simulink model "DriveCtrlModeBase2012"  (R2012a)
settings: Solver=FixedStepDiscrete  SolverMode=SingleTasking  StartTime=0.0  StopTime=10.0  FixedStep=1e-4  RelTol=1e-3
settings Model: CovMetricSettings=dwe  CovHtmlReporting=off  covSaveCumulativeToWorkspaceVar=off  CovSaveSingleToWorkspaceVar=off  CovExternalEMLEnable=on  Creator=F001456D  LastModifiedBy=C000874D
settings DataIOCC: SaveFormat=StructureWithTime  ReturnWorkspaceOutputs=off
settings OptimizationCC: LifeSpan=inf  SimCompilerOptimization=Off
settings DebuggingCC: InheritedTsInSrcMsg=none  FcnCallInpInsideContextMsg=Enable All  RootOutportRequireBusObject=error  StrictBusMsg=ErrorOnBusTreatedAsVector
settings HardwareCC: ProdBitPerPointer=32  ProdLargestAtomicInteger=Long  ProdWordSize=32  ProdHWDeviceType=ARM Compatible->ARM 7
settings SFSimCC: SimUseLocalCustomCode=off
settings RTWCC: SystemTargetFile=MTRealTime_ZYNQ.tlc  TemplateMakefile=MTRealTime_ZYNQ.tmf  Description=MT RealTime ZYNQ Target  RTWUseLocalCustomCode=off  RTWCompilerOptimization=Off
settings STFCustomTargetCC: CodeReplacementLibrary=C99 (ISO)  SystemTargetFile=MTRealTime_ZYNQ.tlc
settings GRTTargetCC: CodeReplacementLibrary=C99 (ISO)  ParMdlRefBuildCompliant=off  CompOptLevelCompliant=off  ConcurrentExecutionCompliant=off  CombineOutputUpdateFcns=off  MatFileLogging=off  CPPClassGenCompliant=off  GRTInterface=on
settings SimscapeCC: SimscapeNormalizeSystem=off

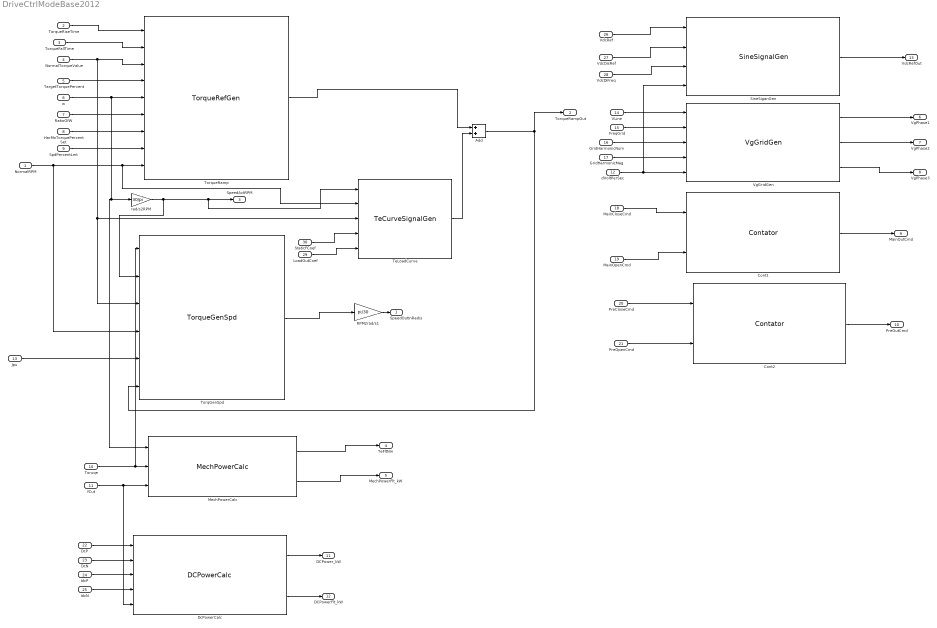
== system DriveCtrlModeBase2012 ==
  NormalRPM : Inport
  TorqueRiseTime : Inport  Port=2
  TorqueFallTime : Inport  Port=3
  NormalTorqueValue : Inport  Port=4
  TargetTorquePercent : Inport  Port=5
  w : Inport  Port=6
  RatioOfW : Inport  Port=7
  HarMoTorquePercentSet : Inport  Port=8
  SpdPercentLmt : Inport  Port=9
  Toruqe : Inport  Port=10
  fCut : Inport  Port=11
  dVoltPerSec : Inport  Port=12
  Jpu : Inport  Port=13
  VLine : Inport  Port=14
  FreqGrid : Inport  Port=15
  GridHarmonicNum : Inport  Port=16
  GridHarmonicMag : Inport  Port=17
  MainCloseCmd : Inport  Port=18
  MainOpenCmd : Inport  Port=19
  PreCloseCmd : Inport  Port=20
  PreOpenCmd : Inport  Port=21
  DcP : Inport  Port=22
  DcN : Inport  Port=23
  IdcP : Inport  Port=24
  IdcN : Inport  Port=25
  VdcRef : Inport  Port=26
  VdcDisRef : Inport  Port=27
  VdcDiFreq : Inport  Port=28
  LoadOutCoef : Inport  Port=29
  StaticFCoef : Inport  Port=30
  Add : Sum
  Cont1 : S-Function  InitFcn=try, set_param(gcb,'FunctionName','Contator'), end  FunctionName=Contator  SFunctionModules=Contator_wrapper  SFunctionDeploymentMode=off  EnableBusSupport=off  mask(S-Function Builder){}
      mask help: Simulink:masks:SFunctionBuilder_MD
      mask init:
      | val = [[.9  0.75 0.75 1 1 .9 .9 1]',[1 1 0.75 0.75 .9 .9 1 .9]'];try , sys = get_param(gcb,'SfunBuilderFcnName');if isempty(sys), sys = get_param(gcb,'FunctionName'); end,catch, sys = get_param(gcb,'FunctionName'); end
      settings: CopyFcn=set_param(gcbh,'LinkStatus','none')  PreSaveFcn=try, set_param(gcb,'FunctionName','Contator'), end  OpenFcn=sfunctionwizard(gcbh)
      mask Display: plot(val(:,1),val(:,2)),disp(sys), port_label('input',1,'CloseCmd'), port_label('input',2,'OpenCmd'), port_label('output',1,'ConCmd')
  Cont2 : S-Function  InitFcn=try, set_param(gcb,'FunctionName','Contator'), end  FunctionName=Contator  SFunctionModules=Contator_wrapper  SFunctionDeploymentMode=off  EnableBusSupport=off  mask(S-Function Builder){}
      mask help: Simulink:masks:SFunctionBuilder_MD
      mask init: same as DriveCtrlModeBase2012/Cont1
      settings: CopyFcn=set_param(gcbh,'LinkStatus','none')  PreSaveFcn=try, set_param(gcb,'FunctionName','Contator'), end  OpenFcn=sfunctionwizard(gcbh)
      mask Display: plot(val(:,1),val(:,2)),disp(sys), port_label('input',1,'CloseCmd'), port_label('input',2,'OpenCmd'), port_label('output',1,'ConCmd')
  DcPowerCalc : S-Function  InitFcn=try, set_param(gcb,'FunctionName','DCPowerCalc'), end  FunctionName=DCPowerCalc  SFunctionModules=DCPowerCalc_wrapper  SFunctionDeploymentMode=off  EnableBusSupport=off  mask(S-Function Builder){}
      mask help: Simulink:masks:SFunctionBuilder_MD
      mask init: same as DriveCtrlModeBase2012/Cont1
      settings: CopyFcn=set_param(gcbh,'LinkStatus','none')  PreSaveFcn=try, set_param(gcb,'FunctionName','DCPowerCalc'), end  OpenFcn=sfunctionwizard(gcbh)
      mask Display: plot(val(:,1),val(:,2)),disp(sys), port_label('input',1,'VdcP'), port_label('input',2,'VdcN'), port_label('input',3,'IdcP'), port_label('input',4,'IdcN'), port_label('input',5,'fCut'), port_label('output',1,'DCPower_kW'), port_label('output',2,'DCPowerFlt_kW')
  MechPowerCalc : S-Function  InitFcn=try, set_param(gcb,'FunctionName','MechPowerCalc'), end  FunctionName=MechPowerCalc  SFunctionModules=MechPowerCalc_wrapper  SFunctionDeploymentMode=off  EnableBusSupport=off  mask(S-Function Builder){}
      mask help: Simulink:masks:SFunctionBuilder_MD
      mask init: same as DriveCtrlModeBase2012/Cont1
      settings: CopyFcn=set_param(gcbh,'LinkStatus','none')  PreSaveFcn=try, set_param(gcb,'FunctionName','MechPowerCalc'), end  OpenFcn=sfunctionwizard(gcbh)
      mask Display: plot(val(:,1),val(:,2)),disp(sys), port_label('input',1,'Wm'), port_label('input',2,'Torque'), port_label('input',3,'fCut'), port_label('output',1,'MechPower_kW'), port_label('output',2,'MechPowerFlt_kW')
  RPM2rad/s1 : Gain  Gain=pi/30
  SineSiganGen : S-Function  InitFcn=try, set_param(gcb,'FunctionName','SineSignalGen'), end  FunctionName=SineSignalGen  SFunctionModules=SineSignalGen_wrapper  SFunctionDeploymentMode=off  EnableBusSupport=off  mask(S-Function Builder){}
      mask help: Simulink:masks:SFunctionBuilder_MD
      mask init: same as DriveCtrlModeBase2012/Cont1
      settings: CopyFcn=set_param(gcbh,'LinkStatus','none')  PreSaveFcn=try, set_param(gcb,'FunctionName','SineSignalGen'), end  OpenFcn=sfunctionwizard(gcbh)
      mask Display: plot(val(:,1),val(:,2)),disp(sys), port_label('input',1,'DCMag'), port_label('input',2,'ACMag'), port_label('input',3,'Freq'), port_label('input',4,'dVoltPerSec'), port_label('output',1,'SineOut')
  TeLoadCurve : S-Function  InitFcn=try, set_param(gcb,'FunctionName','TeCurveSignalGen'), end  FunctionName=TeCurveSignalGen  SFunctionModules=TeCurveSignalGen_wrapper  SFunctionDeploymentMode=off  EnableBusSupport=off  mask(S-Function Builder){}
      mask help: Simulink:masks:SFunctionBuilder_MD
      mask init: same as DriveCtrlModeBase2012/Cont1
      settings: CopyFcn=set_param(gcbh,'LinkStatus','none')  PreSaveFcn=try, set_param(gcb,'FunctionName','TeCurveSignalGen'), end  OpenFcn=sfunctionwizard(gcbh)
      mask Display: plot(val(:,1),val(:,2)),disp(sys), port_label('input',1,'nrpm'), port_label('input',2,'NormRpm'), port_label('input',3,'TeNorm'), port_label('input',4,'StaticFCoef'), port_label('input',5,'KpLoadCurve'), port_label('output',1,'TLCurveOut')
  TorqGenSpd : S-Function  InitFcn=try, set_param(gcb,'FunctionName','TorqueGenSpd'), end  FunctionName=TorqueGenSpd  SFunctionModules=TorqueGenSpd_wrapper  SFunctionDeploymentMode=off  EnableBusSupport=off  mask(S-Function Builder){}
      mask help: Simulink:masks:SFunctionBuilder_MD
      mask init: same as DriveCtrlModeBase2012/Cont1
      settings: CopyFcn=set_param(gcbh,'LinkStatus','none')  PreSaveFcn=try, set_param(gcb,'FunctionName','TorqueGenSpd'), end  OpenFcn=sfunctionwizard(gcbh)
      mask Display: plot(val(:,1),val(:,2)),disp(sys), port_label('input',1,'TorqMotor'), port_label('input',2,'SpdAct'), port_label('input',3,'TorqBase'), port_label('input',4,'SpdBase'), port_label('input',5,'Jpu'), port_label('input',6,'TorqLoad'), port_label('output',1,'SpdSetOut')
  TorqueRamp : S-Function  InitFcn=try, set_param(gcb,'FunctionName','TorqueRefGen'), end  FunctionName=TorqueRefGen  SFunctionModules=TorqueRefGen_wrapper  SFunctionDeploymentMode=off  EnableBusSupport=off  mask(S-Function Builder){}
      mask help: Simulink:masks:SFunctionBuilder_MD
      mask init: same as DriveCtrlModeBase2012/Cont1
      settings: CopyFcn=set_param(gcbh,'LinkStatus','none')  PreSaveFcn=try, set_param(gcb,'FunctionName','TorqueRefGen'), end  OpenFcn=sfunctionwizard(gcbh)
      mask Display: plot(val(:,1),val(:,2)),disp(sys), port_label('input',1,'RiseTime'), port_label('input',2,'FallTime'), port_label('input',3,'NormalValue'), port_label('input',4,'DestValuePercent'), port_label('input',5,'w'), port_label('input',6,'RatioOfW'), port_label('input',7,'HarmoTorquePercent'), port_label('input',8,'SpdPercentLmt'), port_label('input',9,'RPMNorm'), port_label('output',1,'RampOut')
  VgGridGen : S-Function  InitFcn=try, set_param(gcb,'FunctionName','VgGridGen'), end  FunctionName=VgGridGen  SFunctionModules=VgGridGen_wrapper  SFunctionDeploymentMode=off  EnableBusSupport=off  mask(S-Function Builder){}
      mask help: Simulink:masks:SFunctionBuilder_MD
      mask init: same as DriveCtrlModeBase2012/Cont1
      settings: CopyFcn=set_param(gcbh,'LinkStatus','none')  PreSaveFcn=try, set_param(gcb,'FunctionName','VgGridGen'), end  OpenFcn=sfunctionwizard(gcbh)
      mask Display: plot(val(:,1),val(:,2)),disp(sys), port_label('input',1,'ACLine'), port_label('input',2,'Freq'), port_label('input',3,'HarmonicNum'), port_label('input',4,'HarmonicMag'), port_label('input',5,'dVoltPerSec'), port_label('output',1,'VgPhaseA'), port_label('output',2,'VgPhaseB'), port_label('output',3,'VgPhaseC')
  rad/s2RPM : Gain  Gain=30/pi
  SpeedOutInRad/s : Outport
  TorqueRampOut : Outport  Port=2
  SpeedActRPM : Outport  Port=3
  TeFltNm : Outport  Port=4
  MechPowerFlt_kW : Outport  Port=5
  VgPhase1 : Outport  Port=6
  VgPhase2 : Outport  Port=7
  VgPhase3 : Outport  Port=8
  MainOutCmd : Outport  Port=9
  PreOutCmd : Outport  Port=10
  DCPower_kW : Outport  Port=11
  DCPowerFlt_kW : Outport  Port=12
  VdcRefOut : Outport  Port=13
  wires:
  NormalRPM/1 -> TorqGenSpd/4, TeLoadCurve/2, TorqueRamp/9
  rad/s2RPM/1 -> TeLoadCurve/1, SpeedActRPM/1, TorqGenSpd/2
  MechPowerCalc/1 -> TeFltNm/1
  MechPowerCalc/2 -> MechPowerFlt_kW/1
  Toruqe/1 -> MechPowerCalc/2, TorqGenSpd/1
  SpdPercentLmt/1 -> TorqueRamp/8
  TorqueRiseTime/1 -> TorqueRamp/1
  w/1 -> TorqueRamp/5, rad/s2RPM/1, MechPowerCalc/1
  HarMoTorquePercentSet/1 -> TorqueRamp/7
  TargetTorquePercent/1 -> TorqueRamp/4
  RatioOfW/1 -> TorqueRamp/6
  TorqueFallTime/1 -> TorqueRamp/2
  NormalTorqueValue/1 -> TorqueRamp/3, TorqGenSpd/3, TeLoadCurve/3
  TorqGenSpd/1 -> RPM2rad/s1/1
  RPM2rad/s1/1 -> SpeedOutInRad/s/1
  Jpu/1 -> TorqGenSpd/5
  MainOpenCmd/1 -> Cont1/2
  Cont2/1 -> PreOutCmd/1
  Cont1/1 -> MainOutCmd/1
  PreOpenCmd/1 -> Cont2/2
  PreCloseCmd/1 -> Cont2/1
  VgGridGen/1 -> VgPhase1/1
  VgGridGen/2 -> VgPhase2/1
  VLine/1 -> VgGridGen/1
  VgGridGen/3 -> VgPhase3/1
  MainCloseCmd/1 -> Cont1/1
  FreqGrid/1 -> VgGridGen/2
  GridHarmonicNum/1 -> VgGridGen/3
  fCut/1 -> DcPowerCalc/5, MechPowerCalc/3
  IdcP/1 -> DcPowerCalc/3
  IdcN/1 -> DcPowerCalc/4
  DcN/1 -> DcPowerCalc/2
  DcP/1 -> DcPowerCalc/1
  DcPowerCalc/1 -> DCPower_kW/1
  DcPowerCalc/2 -> DCPowerFlt_kW/1
  GridHarmonicMag/1 -> VgGridGen/4
  VdcDiFreq/1 -> SineSiganGen/3
  dVoltPerSec/1 -> SineSiganGen/4, VgGridGen/5
  SineSiganGen/1 -> VdcRefOut/1
  VdcRef/1 -> SineSiganGen/1
  VdcDisRef/1 -> SineSiganGen/2
  Add/1 -> TorqueRampOut/1, TorqGenSpd/6
  TorqueRamp/1 -> Add/1
  LoadOutCoef/1 -> TeLoadCurve/5
  StaticFCoef/1 -> TeLoadCurve/4
  TeLoadCurve/1 -> Add/2
